simulink model "test1_stateflow"  (R2017b)
settings: Solver=VariableStepAuto  StartTime=0.0  StopTime=inf  RelTol=1e-3
settings Model: Creator=Bijan  LastModifiedBy=Bijan

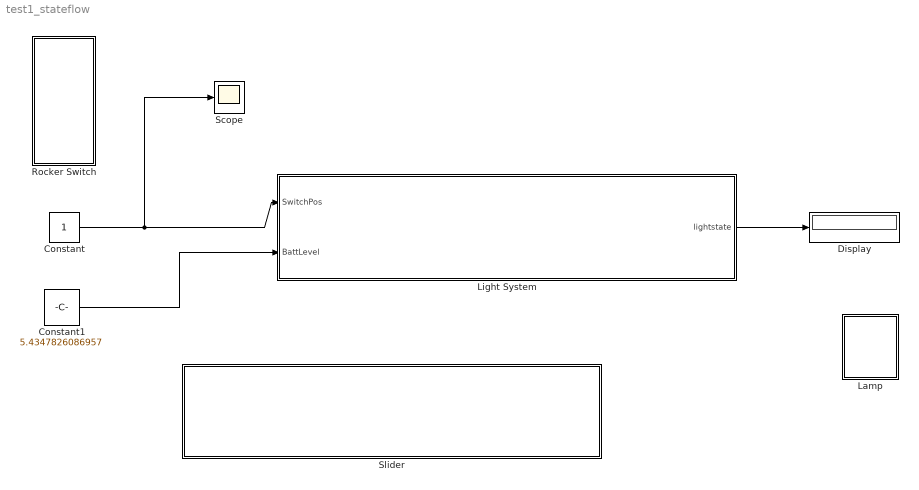
== system test1_stateflow ==
  Constant : Constant
  Constant1 : Constant  Value=5.4347826086957
  Display : Display
  Lamp : Subsystem  DialogController=hmiCreateDDGDialog  IsWebBlock=on  mask(MWDashboardBlock){webBlockId=ecfaaab7-7556-4649-88d9-2a3a5469140d, webBlockType=lamp, ShowInLibBrowser=on, ShowInitialText=on, HMISrcModelName=test1_stateflow}
      mask prompts: webBlockType "WebBlock Type"; HMISrcModelName "Source Model"
      mask help: SimulinkHMI:dialogs:LampDialogDesc
      mask Help: helpview([docroot '/mapfiles/simulink.map'], 'hmi_lamp')
      mask Display:
      | if strcmp(get_param(bdroot(gcb),'BlockDiagramType'), 'library')
      |     image([(matlabroot) '/toolbox/simulink/hmi/icons/Lamp.png']);
      | end
  Light System : Stateflow chart  TreatAsAtomicUnit=on
  Rocker Switch : Subsystem  DialogController=hmiCreateDDGDialog  IsWebBlock=on  mask(MWDashboardBlock){webBlockId=7f899b22-4c87-4d8f-a509-08b9590addb8, webBlockType=rockerswitch, ShowInLibBrowser=on, ShowInitialText=on, HMISrcModelName=test1_stateflow}
      mask prompts: webBlockId "WebBlock Id"; webBlockType "WebBlock Type"; HMISrcModelName "Source Model"
      mask help: SimulinkHMI:dialogs:SwitchDialogDesc
      mask Help: helpview([docroot '/mapfiles/simulink.map'], 'hmi_rocker_switch')
      mask Display:
      | if strcmp(get_param(bdroot(gcb),'BlockDiagramType'), 'library')
      |     image([(matlabroot) '/toolbox/simulink/hmi/icons/RockerSwitch.png']);
      | end
  Scope : Scope
  Slider : Subsystem  DialogController=hmiCreateDDGDialog  IsWebBlock=on  mask(MWDashboardBlock){webBlockId=82c72cf6-5e02-4fcd-9dda-61f4daef99dd, webBlockType=slider, ShowInLibBrowser=on, ShowInitialText=on, HMISrcModelName=test1_stateflow}
      mask prompts: webBlockId "WebBlock Id"; webBlockType "WebBlock Type"; HMISrcModelName "Source Model"
      mask help: SimulinkHMI:dialogs:SliderDialogDesc
      mask Help: helpview([docroot '/mapfiles/simulink.map'], 'hmi_slider')
      mask Display:
      | if strcmp(get_param(bdroot(gcb),'BlockDiagramType'), 'library')
      |     image([(matlabroot) '/toolbox/simulink/hmi/icons/Slider.png']);
      | end
  wires:
  Constant/1 -> Scope/1, Light System/1(SwitchPos)
  Light System/1(lightstate) -> Display/1
  Constant1/1 -> Light System/2(BattLevel)

== system test1_stateflow/Lamp ==

== system test1_stateflow/Rocker Switch ==

== system test1_stateflow/Slider ==

== stateflow chart test1_stateflow/Light System ==
  state OFF
    entry:
    lightstate=0;
  state ON
    entry:
    lightstate=1;
  state Low_Battery
    entry: lightstate=2;
  (default) -> OFF
  OFF -> ON : [SwitchPos==1 && BattLevel>10]
  ON -> OFF [order 1] : [SwitchPos==0]
  Low_Battery -> OFF : [after(10,sec)]
  ON -> Low_Battery [order 2] : [BattLevel<10]
  data: SwitchPos input; lightstate output; BattLevel input
